simulink model "Problem_7"  (R2020a)
settings: Solver=VariableStepAuto  StartTime=0.0  StopTime=10.0  RelTol=1e-3
settings Model: Creator=hp  LastModifiedBy=hp

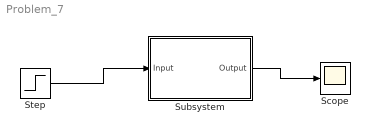
== system Problem_7 ==
  Scope : Scope
  Step : Step  SampleTime=0
  Subsystem : Subsystem
  wires:
  Step/1 -> Subsystem/1(Input)
  Subsystem/1(Output) -> Scope/1

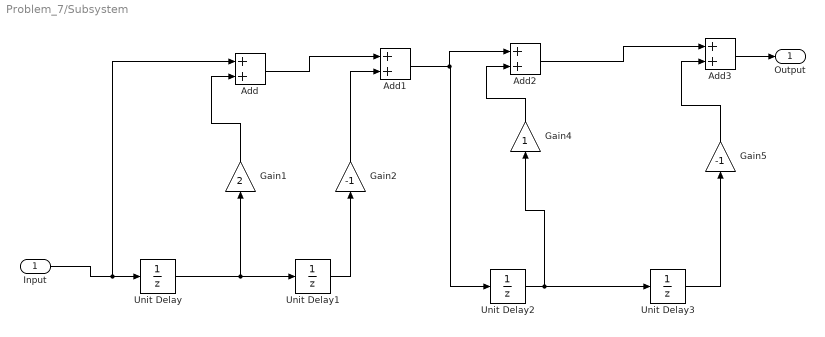
== system Problem_7/Subsystem ==
  Input : Inport
  Add{,1..3} (4 alike) : Sum
  Gain1 : Gain  Gain=2
  Gain2 : Gain  Gain=-1
  Gain4 : Gain
  Gain5 : Gain  Gain=-1
  Unit Delay{,1..3} (4 alike) : UnitDelay  SampleTime=-1  HasFrameUpgradeWarning=on
  Output : Outport
  wires:
  Add3/1 -> Output/1
  Unit Delay/1 -> Gain1/1, Unit Delay1/1
  Unit Delay1/1 -> Gain2/1
  Gain1/1 -> Add/2
  Input/1 -> Add/1, Unit Delay/1
  Gain2/1 -> Add1/2
  Add/1 -> Add1/1
  Add1/1 -> Add2/1, Unit Delay2/1
  Unit Delay2/1 -> Gain4/1, Unit Delay3/1
  Unit Delay3/1 -> Gain5/1
  Gain4/1 -> Add2/2
  Add2/1 -> Add3/1
  Gain5/1 -> Add3/2
